simulink model "skeleton"  (Simulink 5.0)
settings: Solver=ode5  StartTime=0.0  StopTime=10.0  FixedStep=0.001  RelTol=1e-3
libraries: simulink x1
settings Model: Creator=riccardo  LastModifiedBy=riccardo  ExtModeAutoUpdateStatusClock=off  RTWExpressionDepthLimit=0  SaveTime=off  SaveOutput=off  LimitDataPoints=off  RTWInlineParameters=on  RTWSystemTargetFile=ErikaEducational.tlc  RTWTemplateMakefile=ErikaEducational.tmf  RTWRetainRTWFile=on  RTWOptions="-aDOWNLCOMM=\"firmdl\" -aDebugLcd=0 -aDownloadToRobot=0 -aERIKABASE=\"/home/riccardo/erika\" -aEnforceIntegerDowncast=0 -aFoldNonRolledExpr=0 -aForceParamTrailComments=0 -aGenerateComments=1 -aGenerateReport=0 -aH8RTWLIBDIR=\"/home/riccardo/erika/toolbox\" -aIncDataTypeInIds=0 -aIncHierarchyInIds=0 -aInlineInvariantSignals=0 -aInlinedPrmAccess=\"Literals\" -aLEGOTOWERDEVICE=\"/dev/usb/lego0\" -aLocalBlockOutputs=0 -aMaxRTWIdLen=255 -aPrefixModelToSubsysFcnNames=1 -aRTNONFINITE=0 -aRTWVerbose=1 -aRollThreshold=5 -aShowEliminatedStatements=0 -aTaskCF=0 -aUSECUSTCOMM=0 -aUseERT=0 -aVarProcTask=0"

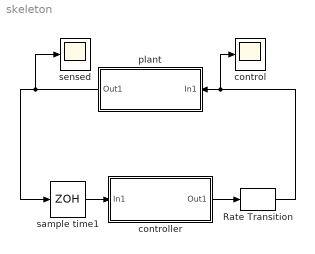
== system skeleton ==
  Rate Transition : simulink/Signal Attributes/Rate Transition  DataIntegrity=on  DeterministicTransfer=on  TransitionType=Slow to fast  InitCond=0
  control : Scope
  controller : Subsystem
  plant : Subsystem  Orientation=left
  sample time1 : ZeroOrderHold  SampleTime=0.1
      settings: AttributesFormatString=%<SampleTime>
  sensed : Scope
  wires:
  plant/1(Out1) -> sample time1/1, sensed/1
  controller/1(Out1) -> Rate Transition/1
  sample time1/1 -> controller/1(In1)
  Rate Transition/1 -> plant/1(In1), control/1

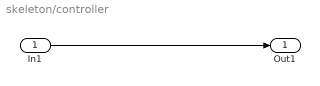
== system skeleton/controller ==
  In1 : Inport
  Out1 : Outport
  wires:
  In1/1 -> Out1/1

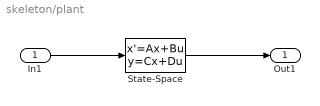
== system skeleton/plant ==
  In1 : Inport
  State-Space : StateSpace
  Out1 : Outport
  wires:
  In1/1 -> State-Space/1
  State-Space/1 -> Out1/1
